simulink model "VehicleSteering_sim_Int"  (Simulink 8.4)
settings: Solver=ode45  SolverMode=SingleTasking  StartTime=0.0  StopTime=10.0  RelTol=1e-3
values from neighbouring files (symbols this model uses):
  A = [0 v0;0 0]    [Example_VehicleSteering_Integral_action.m]    (also in Example_VehicleSteering_LQR.m; Example_VehicleSteering_SS_control.m)
  B = [a*v0/b v0/b]'    [Example_VehicleSteering_Integral_action.m]    (also in Example_VehicleSteering_LQR.m; Example_VehicleSteering_SS_control.m)
  C = eye(2)    [Example_VehicleSteering_Integral_action.m]    (also in Example_VehicleSteering_LQR.m; Example_VehicleSteering_SS_control.m)
  D = [0 0]'    [Example_VehicleSteering_Integral_action.m]    (also in Example_VehicleSteering_LQR.m; Example_VehicleSteering_SS_control.m)
  Ku = (p - ap) * Wr_tilde * Wr^(-1)    [Example_VehicleSteering_Integral_action.m]
settings Model: Creator=jofr  LastModifiedBy=rodralez  CovMetricSettings=dwe  CovHtmlReporting=off  covSaveCumulativeToWorkspaceVar=off  CovSaveSingleToWorkspaceVar=off  CovExternalEMLEnable=on  CovSFcnEnable=on
settings DataIOCC: LimitDataPoints=off  SaveFormat=StructureWithTime  SignalLoggingSaveFormat=Dataset
settings OptimizationCC: ExpressionDepthLimit=128
settings DebuggingCC: UnderspecifiedInitializationDetection=Simplified  MergeDetectMultiDrivingBlocksExec=error  SolverPrmCheckMsg=none  FcnCallInpInsideContextMsg=EnableAllAsError  FrameProcessingCompatibilityMsg=error  StateNameClashWarn=none  SFUnexpectedBacktrackingDiag=error  SFNoUnconditionalDefaultTransitionDiag=error
settings HardwareCC: ProdBitPerPointer=64  ProdLargestAtomicFloat=Float  ProdIntDivRoundTo=Zero  ProdEndianess=LittleEndian  ProdHWDeviceType=Specified
settings ModelReferenceCC: PropagateSignalLabelsOutOfModel=on
settings GRTTargetCC: TargetLangStandard=C99 (ISO)  CombineOutputUpdateFcns=on  GRTInterface=off

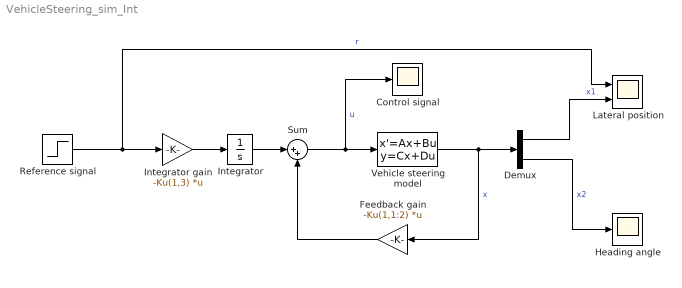
== system VehicleSteering_sim_Int ==
  Control signal : Scope
      settings: TimeRange=auto  MaxDataPoints=5000  SaveName=u  YMin=-0.0077  YMax=0.03172  SampleTime=-1  DataFormat=Array
  Demux : Demux  Outputs=2
  Feedback gain : Gain  Gain=-Ku(1,1:2)  Multiplication=Matrix(K*u)
  Heading angle : Scope
      settings: TimeRange=auto  MaxDataPoints=5000  SaveName=x2  YMin=-0.02563  YMax=0.23068  SampleTime=-1
  Integrator : Integrator
  Integrator gain : Gain  Gain=-Ku(1,3)  Multiplication=Matrix(K*u)
  Lateral position : Scope  NumInputPorts=2
      settings: TimeRange=auto  MaxDataPoints=5000  SaveName=x1  YMin=-8.85475~-5  YMax=79.69273~5  SampleTime=-1
  "Reference signal " : Step  SampleTime=0
  Sum : Sum  Inputs=|++
  Vehicle steering model : StateSpace  A=A  B=B  C=C  D=D  X0=0
  wires:
  Vehicle steering model/1 -> Demux/1, Feedback gain/1  "x"
  Sum/1 -> Control signal/1, Vehicle steering model/1  "u"
  Feedback gain/1 -> Sum/2
  Demux/2 -> Heading angle/1  "x2"
  "Reference signal "/1 -> Integrator gain/1, Lateral position/1  "r"
  Demux/1 -> Lateral position/2  "x1"
  Integrator gain/1 -> Integrator/1
  Integrator/1 -> Sum/1
